simulink model "asynchronous_motor_rpm"  (R2017b)
settings: Solver=VariableStepAuto  StartTime=0.0  StopTime=10.0  MaxStep=1e-4  RelTol=1e-3
libraries: powerlib x3
settings Model: Creator=Damla  LastModifiedBy=dagac

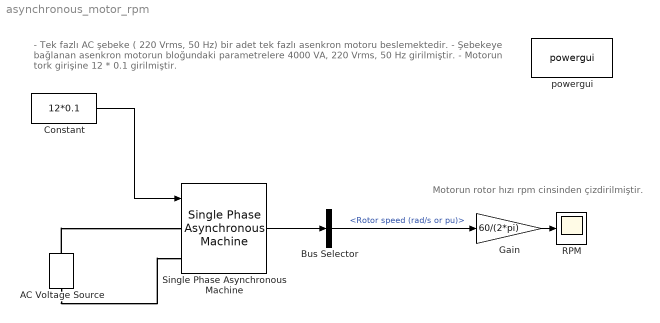
== system asynchronous_motor_rpm ==
  note: Motorun rotor hızı rpm cinsinden çizdirilmiştir.
  note: - Tek fazlı AC şebeke ( 220 Vrms, 50 Hz) bir adet tek fazlı asenkron motoru beslemektedir.
      | - Şebekeye bağlanan asenkron motorun bloğundaki parametrelere 4000 VA, 220 Vrms, 50 Hz girilmiştir.
      | - Motorun tork girişine 12 * 0.1 girilmiştir.
  AC Voltage Source : powerlib/Electrical Sources/AC Voltage Source  Amplitude=311.12  Phase=0  Frequency=50  SampleTime=0  Measurements=None  BusType=swing  Pref=10e3  Qref=0  Qmin=-inf  Qmax=+inf
  Bus Selector : BusSelector  OutputSignals=Mechanical.Rotor speed (rad/s or pu)
  Constant : Constant  Value=12*0.1
  Gain : Gain  Gain=60/(2*pi)
  RPM : Scope
  Single Phase Asynchronous Machine : powerlib/Machines/Single Phase Asynchronous Machine  MechanicalLoad=Torque Tm  UNITS=SI  MachineType=Split Phase  MeasurementBus=off  NominalParameters="[ 4000  220  50]"  MainWindingStator="[2.02  7.4e-3]"  MainWindingRotor="[4.12  5.6e-3]"  MutualInductance=0.1772  AuxiliaryWinding="[7.14  8.5e-3]"  Mechanical="[0.0146  0  2 1.18]"  CapacitorStart="[2  254.7e-6]"  CapacitorRun="[18  21.1e-6]"  DisconnectionSpeed=75  InitialSpeed=0  DataType=SI  TsPowergui=0  TsBlock=-1
      settings: SourceProductName=Simscape Power Systems  SourceProductBaseCode=PS
  powergui : powerlib/powergui  Priority=1  SimulationMode=Continuous  SampleTime=50e-6  frequency=60  Iterations=50  frequencyindice=50  Pbase=100e6  ErrMax=1e-4  UnitsV=kV  UnitsW=MW  buscounter=0  FunctionMessages=off  echomessages=off  EnableUseOfTLC=off  CurrentSourceSwitches=off  DisableSnubberDevices=off  DisableRonSwitches=off  DisableVfSwitches=off  DisplayEquations=off  SolverType=Tustin/Backward Euler (TBE)  Interpol=off  ExternalGateDelay=off  methode=off  Ts=100  x0status=blocks  SPID=on  SwTol=0  HookPort=off  RestoreLinks=warning  ResistiveCurrentMeasurement=off  Frange=[0:2:500]  Ylog=off  Xlog=on  ShowGrid=off  save=off  variable=ZData  structure=0  ZoomFFT=off  StartTime=0.0  cycles=1  DisplayStyle=1  fundamental=60  FreqAxis=off  MaxFrequency=1000  frequencyindicesteady=1  RmsSteady=1  display=off
  wires:
  Single Phase Asynchronous Machine/1 -> Bus Selector/1
  Constant/1 -> Single Phase Asynchronous Machine/1
  Bus Selector/1 -> Gain/1  "<Rotor speed (rad/s or pu)>"
  Gain/1 -> RPM/1
  connections:
  AC Voltage Source/LConn1 -- Single Phase Asynchronous Machine/LConn2
  AC Voltage Source/RConn1 -- Single Phase Asynchronous Machine/LConn1
